simulink model "control_path"  (R2020b)
settings: Solver=FixedStepDiscrete  StartTime=0.0  StopTime=stopTime  FixedStep=2.0833333333333333e-05  RelTol=1e-3
settings Model: Creator=Ross  LastModifiedBy=tyler
settings DataIOCC: SaveOutput=off  SaveTime=off  ReturnWorkspaceOutputs=off
settings OptimizationCC: BlockReduction=off  ConditionallyExecuteInputs=off  DefaultParameterBehavior=Inlined
settings DebuggingCC: ReadBeforeWriteMsg=DisableAll  WriteAfterWriteMsg=DisableAll  WriteAfterReadMsg=DisableAll  AlgebraicLoopMsg=error  MultiTaskDSMMsg=none  SingleTaskRateTransMsg=error  PregeneratedLibrarySubsystemCodeDiagnostic=none  ArithmeticOperatorsInVariantConditions=warning
settings HardwareCC: ProdBitPerPointer=32  ProdBitPerSizeT=32  ProdBitPerPtrDiffT=32  ProdLargestAtomicFloat=None  ProdIntDivRoundTo=Undefined  ProdEndianess=Unspecified  ProdWordSize=32  ProdHWDeviceType=ASIC/FPGA->ASIC/FPGA  TargetBitPerPointer=64  TargetBitPerSizeT=64  TargetBitPerPtrDiffT=64  TargetLongLongMode=on  TargetIntDivRoundTo=Zero  TargetEndianess=LittleEndian  TargetWordSize=64  TargetHWDeviceType=Custom Processor->MATLAB Host Computer  ProdEqTarget=off
settings ModelReferenceCC: UpdateModelReferenceTargets=IfOutOfDate  ModelReferenceNumInstancesAllowed=Single
settings SFSimCC: SFSimEcho=off  SimUseLocalCustomCode=off  CustomCodeUndefinedFunction=UseInterfaceOnly
settings RTWCC: RTWUseLocalCustomCode=off

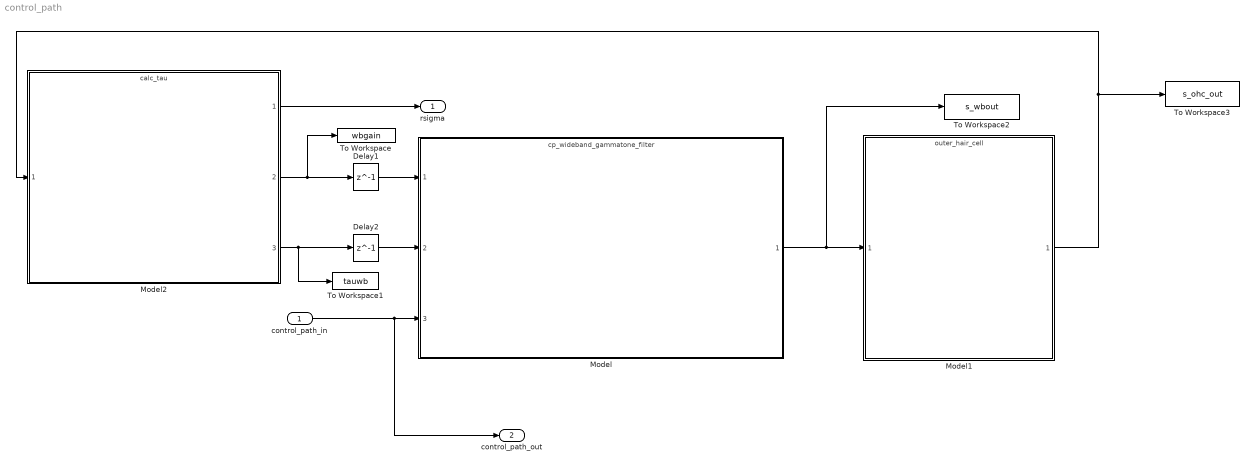
== system control_path ==
  control_path_in : Inport  OutDataTypeStr=single  PortDimensions=1  SampleTime=[2.0833333333333333e-05,0]
  Delay1 : Delay  DelayLength=1  InitialCondition=0  UseCircularBuffer=on
  Delay2 : Delay  DelayLength=1  InitialCondition=0  UseCircularBuffer=on
  Model : ModelReference  ModelNameDialog=cp_wideband_gammatone_filter.slx  SimulationMode=Normal  ModelReferenceVersion=1.124
  Model1 : ModelReference  ModelNameDialog=outer_hair_cell.slx  SimulationMode=Normal  ModelReferenceVersion=1.127
  Model2 : ModelReference  ModelNameDialog=calc_tau.slx  SimulationMode=Normal  ModelReferenceVersion=1.132
  To Workspace : ToWorkspace  VariableName=wbgain  SampleTime=-1
  To Workspace1 : ToWorkspace  VariableName=tauwb  SampleTime=-1
  To Workspace2 : ToWorkspace  VariableName=s_wbout  SampleTime=-1
  To Workspace3 : ToWorkspace  VariableName=s_ohc_out  SampleTime=-1
  rsigma : Outport  OutDataTypeStr=single  PortDimensions=1  SampleTime=[2.0833333333333333e-05,0]
  control_path_out : Outport  Port=2  OutDataTypeStr=single  PortDimensions=1  SampleTime=[2.0833333333333333e-05,0]
  wires:
  Model2/3 -> Delay2/1, To Workspace1/1
  Model2/2 -> Delay1/1, To Workspace/1
  Model1/1 -> Model2/1, To Workspace3/1
  Model/1 -> Model1/1, To Workspace2/1
  Model2/1 -> rsigma/1
  control_path_in/1 -> control_path_out/1, Model/3
  Delay1/1 -> Model/1
  Delay2/1 -> Model/2
